simulink model "ROBOT_OK"  (R2021a)
settings: Solver=FixedStepAuto  StartTime=0.0  StopTime=inf  FixedStep=0.001  RelTol=1e-3
model workspace: external: MATLAB File E:\2024\TINH_TOAN_ROBOT_6_DOF\ROBOT_OK_DataFile.m (data not in the file)
values from neighbouring files (symbols this model uses):
  X = Toado(:,1)    [QuydaoK.m]
  Y = Toado(:,2)    [QuydaoK.m]
  Z = Toado(:,3)    [QuydaoK.m]
undefined symbols (not defined in the file or in its folder): smiData
libraries: sm_lib x38, nesl_utility x30, sharedutil x16, sharedtransform x12, dspmtrx3 x12, simulink_extras x8, pid_lib x6, simulink x3
(part 5 of 6)

== system ROBOT_OK/Subsystem2/Jacobian/J(q) gen./J_v_3(q)/J_v_1 ==
  R : Inport
  p : Inport  Port=2
  pn : Inport  Port=3
  type : Inport  Port=4
  Add : Sum
  If : If  IfExpression=u1 == 1
  Prismatic Action : Subsystem  TreatAsAtomicUnit=on
  Revolute Action : Subsystem  TreatAsAtomicUnit=on
  J_v : Outport
  wires:
  type/1 -> If/1
  If/1 -> Revolute Action/Action
  If/2 -> Prismatic Action/Action
  Revolute Action/1(J_v) -> Add/1
  Prismatic Action/1(J_v) -> Add/2
  Add/1 -> J_v/1
  R/1 -> Prismatic Action/1(R), Revolute Action/1(R)
  p/1 -> Revolute Action/2(p)
  pn/1 -> Revolute Action/3(pn)

== system ROBOT_OK/Subsystem2/Jacobian/J(q) gen./J_v_3(q)/J_v_2 ==
  R : Inport
  p : Inport  Port=2
  pn : Inport  Port=3
  type : Inport  Port=4
  Add : Sum
  If : If  IfExpression=u1 == 1
  Prismatic Action : Subsystem  TreatAsAtomicUnit=on
  Revolute Action : Subsystem  TreatAsAtomicUnit=on
  J_v : Outport
  wires:
  type/1 -> If/1
  If/1 -> Revolute Action/Action
  If/2 -> Prismatic Action/Action
  Revolute Action/1(J_v) -> Add/1
  Prismatic Action/1(J_v) -> Add/2
  Add/1 -> J_v/1
  R/1 -> Prismatic Action/1(R), Revolute Action/1(R)
  p/1 -> Revolute Action/2(p)
  pn/1 -> Revolute Action/3(pn)

== system ROBOT_OK/Subsystem2/Jacobian/J(q) gen./J_v_4(q)/J_v_1 ==
  R : Inport
  p : Inport  Port=2
  pn : Inport  Port=3
  type : Inport  Port=4
  Add : Sum
  If : If  IfExpression=u1 == 1
  Prismatic Action : Subsystem  TreatAsAtomicUnit=on
  Revolute Action : Subsystem  TreatAsAtomicUnit=on
  J_v : Outport
  wires:
  type/1 -> If/1
  If/1 -> Revolute Action/Action
  If/2 -> Prismatic Action/Action
  Revolute Action/1(J_v) -> Add/1
  Prismatic Action/1(J_v) -> Add/2
  Add/1 -> J_v/1
  R/1 -> Prismatic Action/1(R), Revolute Action/1(R)
  p/1 -> Revolute Action/2(p)
  pn/1 -> Revolute Action/3(pn)

== system ROBOT_OK/Subsystem2/Jacobian/J(q) gen./J_v_4(q)/J_v_2 ==
  R : Inport
  p : Inport  Port=2
  pn : Inport  Port=3
  type : Inport  Port=4
  Add : Sum
  If : If  IfExpression=u1 == 1
  Prismatic Action : Subsystem  TreatAsAtomicUnit=on
  Revolute Action : Subsystem  TreatAsAtomicUnit=on
  J_v : Outport
  wires:
  type/1 -> If/1
  If/1 -> Revolute Action/Action
  If/2 -> Prismatic Action/Action
  Revolute Action/1(J_v) -> Add/1
  Prismatic Action/1(J_v) -> Add/2
  Add/1 -> J_v/1
  R/1 -> Prismatic Action/1(R), Revolute Action/1(R)
  p/1 -> Revolute Action/2(p)
  pn/1 -> Revolute Action/3(pn)

== system ROBOT_OK/Subsystem2/Jacobian/J(q) gen./J_v_4(q)/J_v_3 ==
  R : Inport
  p : Inport  Port=2
  pn : Inport  Port=3
  type : Inport  Port=4
  Add : Sum
  If : If  IfExpression=u1 == 1
  Prismatic Action : Subsystem  TreatAsAtomicUnit=on
  Revolute Action : Subsystem  TreatAsAtomicUnit=on
  J_v : Outport
  wires:
  type/1 -> If/1
  If/1 -> Revolute Action/Action
  If/2 -> Prismatic Action/Action
  Revolute Action/1(J_v) -> Add/1
  Prismatic Action/1(J_v) -> Add/2
  Add/1 -> J_v/1
  R/1 -> Prismatic Action/1(R), Revolute Action/1(R)
  p/1 -> Revolute Action/2(p)
  pn/1 -> Revolute Action/3(pn)

== system ROBOT_OK/Subsystem2/Jacobian/J(q) gen./J_v_5(q)/J_v_1 ==
  R : Inport
  p : Inport  Port=2
  pn : Inport  Port=3
  type : Inport  Port=4
  Add : Sum
  If : If  IfExpression=u1 == 1
  Prismatic Action : Subsystem  TreatAsAtomicUnit=on
  Revolute Action : Subsystem  TreatAsAtomicUnit=on
  J_v : Outport
  wires:
  type/1 -> If/1
  If/1 -> Revolute Action/Action
  If/2 -> Prismatic Action/Action
  Revolute Action/1(J_v) -> Add/1
  Prismatic Action/1(J_v) -> Add/2
  Add/1 -> J_v/1
  R/1 -> Prismatic Action/1(R), Revolute Action/1(R)
  p/1 -> Revolute Action/2(p)
  pn/1 -> Revolute Action/3(pn)

== system ROBOT_OK/Subsystem2/Jacobian/J(q) gen./J_v_5(q)/J_v_2 ==
  R : Inport
  p : Inport  Port=2
  pn : Inport  Port=3
  type : Inport  Port=4
  Add : Sum
  If : If  IfExpression=u1 == 1
  Prismatic Action : Subsystem  TreatAsAtomicUnit=on
  Revolute Action : Subsystem  TreatAsAtomicUnit=on
  J_v : Outport
  wires:
  type/1 -> If/1
  If/1 -> Revolute Action/Action
  If/2 -> Prismatic Action/Action
  Revolute Action/1(J_v) -> Add/1
  Prismatic Action/1(J_v) -> Add/2
  Add/1 -> J_v/1
  R/1 -> Prismatic Action/1(R), Revolute Action/1(R)
  p/1 -> Revolute Action/2(p)
  pn/1 -> Revolute Action/3(pn)

== system ROBOT_OK/Subsystem2/Jacobian/J(q) gen./J_v_5(q)/J_v_3 ==
  R : Inport
  p : Inport  Port=2
  pn : Inport  Port=3
  type : Inport  Port=4
  Add : Sum
  If : If  IfExpression=u1 == 1
  Prismatic Action : Subsystem  TreatAsAtomicUnit=on
  Revolute Action : Subsystem  TreatAsAtomicUnit=on
  J_v : Outport
  wires:
  type/1 -> If/1
  If/1 -> Revolute Action/Action
  If/2 -> Prismatic Action/Action
  Revolute Action/1(J_v) -> Add/1
  Prismatic Action/1(J_v) -> Add/2
  Add/1 -> J_v/1
  R/1 -> Prismatic Action/1(R), Revolute Action/1(R)
  p/1 -> Revolute Action/2(p)
  pn/1 -> Revolute Action/3(pn)

== system ROBOT_OK/Subsystem2/Jacobian/J(q) gen./J_v_5(q)/J_v_4 ==
  R : Inport
  p : Inport  Port=2
  pn : Inport  Port=3
  type : Inport  Port=4
  Add : Sum
  If : If  IfExpression=u1 == 1
  Prismatic Action : Subsystem  TreatAsAtomicUnit=on
  Revolute Action : Subsystem  TreatAsAtomicUnit=on
  J_v : Outport
  wires:
  type/1 -> If/1
  If/1 -> Revolute Action/Action
  If/2 -> Prismatic Action/Action
  Revolute Action/1(J_v) -> Add/1
  Prismatic Action/1(J_v) -> Add/2
  Add/1 -> J_v/1
  R/1 -> Prismatic Action/1(R), Revolute Action/1(R)
  p/1 -> Revolute Action/2(p)
  pn/1 -> Revolute Action/3(pn)

== system ROBOT_OK/Subsystem2/Jacobian/J_v/J_v_1/Prismatic Action ==
  R : Inport
  Action Port : ActionPort  ActionPortLabel=else
  Constant : Constant  Value=[0;0;1]
  Product : Product  Multiplication=Matrix(*)
  J_v : Outport
  wires:
  Product/1 -> J_v/1
  R/1 -> Product/1
  Constant/1 -> Product/2

== system ROBOT_OK/Subsystem2/Jacobian/J_v/J_v_1/Revolute Action ==
  R : Inport
  p : Inport  Port=2
  pn : Inport  Port=3
  Action Port : ActionPort  ActionPortLabel=if(u1 == 1)
  3x3 Cross Product : sharedutil/3x3 Cross Product  aMode=aMode
      settings: SourceProductBaseCode=AE
  Add : Sum  Inputs=-+
  Constant : Constant  Value=[0;0;1]
  Product : Product  Multiplication=Matrix(*)
  J_v : Outport
  wires:
  3x3 Cross Product/1 -> J_v/1
  p/1 -> Add/1
  pn/1 -> Add/2
  Add/1 -> 3x3 Cross Product/2
  R/1 -> Product/1
  Constant/1 -> Product/2
  Product/1 -> 3x3 Cross Product/1

== system ROBOT_OK/Subsystem2/Jacobian/J_v/J_v_2/Prismatic Action ==
  R : Inport
  Action Port : ActionPort  ActionPortLabel=else
  Constant : Constant  Value=[0;0;1]
  Product : Product  Multiplication=Matrix(*)
  J_v : Outport
  wires:
  Product/1 -> J_v/1
  R/1 -> Product/1
  Constant/1 -> Product/2

== system ROBOT_OK/Subsystem2/Jacobian/J_v/J_v_2/Revolute Action ==
  R : Inport
  p : Inport  Port=2
  pn : Inport  Port=3
  Action Port : ActionPort  ActionPortLabel=if(u1 == 1)
  3x3 Cross Product : sharedutil/3x3 Cross Product  aMode=aMode
      settings: SourceProductBaseCode=AE
  Add : Sum  Inputs=-+
  Constant : Constant  Value=[0;0;1]
  Product : Product  Multiplication=Matrix(*)
  J_v : Outport
  wires:
  3x3 Cross Product/1 -> J_v/1
  p/1 -> Add/1
  pn/1 -> Add/2
  Add/1 -> 3x3 Cross Product/2
  R/1 -> Product/1
  Constant/1 -> Product/2
  Product/1 -> 3x3 Cross Product/1

== system ROBOT_OK/Subsystem2/Jacobian/J_v/J_v_3/Prismatic Action ==
  R : Inport
  Action Port : ActionPort  ActionPortLabel=else
  Constant : Constant  Value=[0;0;1]
  Product : Product  Multiplication=Matrix(*)
  J_v : Outport
  wires:
  Product/1 -> J_v/1
  R/1 -> Product/1
  Constant/1 -> Product/2

== system ROBOT_OK/Subsystem2/Jacobian/J_v/J_v_3/Revolute Action ==
  R : Inport
  p : Inport  Port=2
  pn : Inport  Port=3
  Action Port : ActionPort  ActionPortLabel=if(u1 == 1)
  3x3 Cross Product : sharedutil/3x3 Cross Product  aMode=aMode
      settings: SourceProductBaseCode=AE
  Add : Sum  Inputs=-+
  Constant : Constant  Value=[0;0;1]
  Product : Product  Multiplication=Matrix(*)
  J_v : Outport
  wires:
  3x3 Cross Product/1 -> J_v/1
  p/1 -> Add/1
  pn/1 -> Add/2
  Add/1 -> 3x3 Cross Product/2
  R/1 -> Product/1
  Constant/1 -> Product/2
  Product/1 -> 3x3 Cross Product/1

== system ROBOT_OK/Subsystem2/Jacobian/J_v/J_v_4/Prismatic Action ==
  R : Inport
  Action Port : ActionPort  ActionPortLabel=else
  Constant : Constant  Value=[0;0;1]
  Product : Product  Multiplication=Matrix(*)
  J_v : Outport
  wires:
  Product/1 -> J_v/1
  R/1 -> Product/1
  Constant/1 -> Product/2

== system ROBOT_OK/Subsystem2/Jacobian/J_v/J_v_4/Revolute Action ==
  R : Inport
  p : Inport  Port=2
  pn : Inport  Port=3
  Action Port : ActionPort  ActionPortLabel=if(u1 == 1)
  3x3 Cross Product : sharedutil/3x3 Cross Product  aMode=aMode
      settings: SourceProductBaseCode=AE
  Add : Sum  Inputs=-+
  Constant : Constant  Value=[0;0;1]
  Product : Product  Multiplication=Matrix(*)
  J_v : Outport
  wires:
  3x3 Cross Product/1 -> J_v/1
  p/1 -> Add/1
  pn/1 -> Add/2
  Add/1 -> 3x3 Cross Product/2
  R/1 -> Product/1
  Constant/1 -> Product/2
  Product/1 -> 3x3 Cross Product/1

== system ROBOT_OK/Subsystem2/Jacobian/J_v/J_v_5/Prismatic Action ==
  R : Inport
  Action Port : ActionPort  ActionPortLabel=else
  Constant : Constant  Value=[0;0;1]
  Product : Product  Multiplication=Matrix(*)
  J_v : Outport
  wires:
  Product/1 -> J_v/1
  R/1 -> Product/1
  Constant/1 -> Product/2

== system ROBOT_OK/Subsystem2/Jacobian/J_v/J_v_5/Revolute Action ==
  R : Inport
  p : Inport  Port=2
  pn : Inport  Port=3
  Action Port : ActionPort  ActionPortLabel=if(u1 == 1)
  3x3 Cross Product : sharedutil/3x3 Cross Product  aMode=aMode
      settings: SourceProductBaseCode=AE
  Add : Sum  Inputs=-+
  Constant : Constant  Value=[0;0;1]
  Product : Product  Multiplication=Matrix(*)
  J_v : Outport
  wires:
  3x3 Cross Product/1 -> J_v/1
  p/1 -> Add/1
  pn/1 -> Add/2
  Add/1 -> 3x3 Cross Product/2
  R/1 -> Product/1
  Constant/1 -> Product/2
  Product/1 -> 3x3 Cross Product/1

== system ROBOT_OK/Subsystem2/Jacobian/J_v/J_v_6/Prismatic Action ==
  R : Inport
  Action Port : ActionPort  ActionPortLabel=else
  Constant : Constant  Value=[0;0;1]
  Product : Product  Multiplication=Matrix(*)
  J_v : Outport
  wires:
  Product/1 -> J_v/1
  R/1 -> Product/1
  Constant/1 -> Product/2

== system ROBOT_OK/Subsystem2/Jacobian/J_v/J_v_6/Revolute Action ==
  R : Inport
  p : Inport  Port=2
  pn : Inport  Port=3
  Action Port : ActionPort  ActionPortLabel=if(u1 == 1)
  3x3 Cross Product : sharedutil/3x3 Cross Product  aMode=aMode
      settings: SourceProductBaseCode=AE
  Add : Sum  Inputs=-+
  Constant : Constant  Value=[0;0;1]
  Product : Product  Multiplication=Matrix(*)
  J_v : Outport
  wires:
  3x3 Cross Product/1 -> J_v/1
  p/1 -> Add/1
  pn/1 -> Add/2
  Add/1 -> 3x3 Cross Product/2
  R/1 -> Product/1
  Constant/1 -> Product/2
  Product/1 -> 3x3 Cross Product/1

== system ROBOT_OK/Động Lực Học2/Jacobian/J(q) gen./J_v_2(q)/J_v_1 ==
  R : Inport
  p : Inport  Port=2
  pn : Inport  Port=3
  type : Inport  Port=4
  Add : Sum
  If : If  IfExpression=u1 == 1
  Prismatic Action : Subsystem  TreatAsAtomicUnit=on
  Revolute Action : Subsystem  TreatAsAtomicUnit=on
  J_v : Outport
  wires:
  type/1 -> If/1
  If/1 -> Revolute Action/Action
  If/2 -> Prismatic Action/Action
  Revolute Action/1(J_v) -> Add/1
  Prismatic Action/1(J_v) -> Add/2
  Add/1 -> J_v/1
  R/1 -> Prismatic Action/1(R), Revolute Action/1(R)
  p/1 -> Revolute Action/2(p)
  pn/1 -> Revolute Action/3(pn)

== system ROBOT_OK/Động Lực Học2/Jacobian/J(q) gen./J_v_3(q)/J_v_1 ==
  R : Inport
  p : Inport  Port=2
  pn : Inport  Port=3
  type : Inport  Port=4
  Add : Sum
  If : If  IfExpression=u1 == 1
  Prismatic Action : Subsystem  TreatAsAtomicUnit=on
  Revolute Action : Subsystem  TreatAsAtomicUnit=on
  J_v : Outport
  wires:
  type/1 -> If/1
  If/1 -> Revolute Action/Action
  If/2 -> Prismatic Action/Action
  Revolute Action/1(J_v) -> Add/1
  Prismatic Action/1(J_v) -> Add/2
  Add/1 -> J_v/1
  R/1 -> Prismatic Action/1(R), Revolute Action/1(R)
  p/1 -> Revolute Action/2(p)
  pn/1 -> Revolute Action/3(pn)

== system ROBOT_OK/Động Lực Học2/Jacobian/J(q) gen./J_v_3(q)/J_v_2 ==
  R : Inport
  p : Inport  Port=2
  pn : Inport  Port=3
  type : Inport  Port=4
  Add : Sum
  If : If  IfExpression=u1 == 1
  Prismatic Action : Subsystem  TreatAsAtomicUnit=on
  Revolute Action : Subsystem  TreatAsAtomicUnit=on
  J_v : Outport
  wires:
  type/1 -> If/1
  If/1 -> Revolute Action/Action
  If/2 -> Prismatic Action/Action
  Revolute Action/1(J_v) -> Add/1
  Prismatic Action/1(J_v) -> Add/2
  Add/1 -> J_v/1
  R/1 -> Prismatic Action/1(R), Revolute Action/1(R)
  p/1 -> Revolute Action/2(p)
  pn/1 -> Revolute Action/3(pn)

== system ROBOT_OK/Động Lực Học2/Jacobian/J(q) gen./J_v_4(q)/J_v_1 ==
  R : Inport
  p : Inport  Port=2
  pn : Inport  Port=3
  type : Inport  Port=4
  Add : Sum
  If : If  IfExpression=u1 == 1
  Prismatic Action : Subsystem  TreatAsAtomicUnit=on
  Revolute Action : Subsystem  TreatAsAtomicUnit=on
  J_v : Outport
  wires:
  type/1 -> If/1
  If/1 -> Revolute Action/Action
  If/2 -> Prismatic Action/Action
  Revolute Action/1(J_v) -> Add/1
  Prismatic Action/1(J_v) -> Add/2
  Add/1 -> J_v/1
  R/1 -> Prismatic Action/1(R), Revolute Action/1(R)
  p/1 -> Revolute Action/2(p)
  pn/1 -> Revolute Action/3(pn)

== system ROBOT_OK/Động Lực Học2/Jacobian/J(q) gen./J_v_4(q)/J_v_2 ==
  R : Inport
  p : Inport  Port=2
  pn : Inport  Port=3
  type : Inport  Port=4
  Add : Sum
  If : If  IfExpression=u1 == 1
  Prismatic Action : Subsystem  TreatAsAtomicUnit=on
  Revolute Action : Subsystem  TreatAsAtomicUnit=on
  J_v : Outport
  wires:
  type/1 -> If/1
  If/1 -> Revolute Action/Action
  If/2 -> Prismatic Action/Action
  Revolute Action/1(J_v) -> Add/1
  Prismatic Action/1(J_v) -> Add/2
  Add/1 -> J_v/1
  R/1 -> Prismatic Action/1(R), Revolute Action/1(R)
  p/1 -> Revolute Action/2(p)
  pn/1 -> Revolute Action/3(pn)

== system ROBOT_OK/Động Lực Học2/Jacobian/J(q) gen./J_v_4(q)/J_v_3 ==
  R : Inport
  p : Inport  Port=2
  pn : Inport  Port=3
  type : Inport  Port=4
  Add : Sum
  If : If  IfExpression=u1 == 1
  Prismatic Action : Subsystem  TreatAsAtomicUnit=on
  Revolute Action : Subsystem  TreatAsAtomicUnit=on
  J_v : Outport
  wires:
  type/1 -> If/1
  If/1 -> Revolute Action/Action
  If/2 -> Prismatic Action/Action
  Revolute Action/1(J_v) -> Add/1
  Prismatic Action/1(J_v) -> Add/2
  Add/1 -> J_v/1
  R/1 -> Prismatic Action/1(R), Revolute Action/1(R)
  p/1 -> Revolute Action/2(p)
  pn/1 -> Revolute Action/3(pn)

== system ROBOT_OK/Động Lực Học2/Jacobian/J(q) gen./J_v_5(q)/J_v_1 ==
  R : Inport
  p : Inport  Port=2
  pn : Inport  Port=3
  type : Inport  Port=4
  Add : Sum
  If : If  IfExpression=u1 == 1
  Prismatic Action : Subsystem  TreatAsAtomicUnit=on
  Revolute Action : Subsystem  TreatAsAtomicUnit=on
  J_v : Outport
  wires:
  type/1 -> If/1
  If/1 -> Revolute Action/Action
  If/2 -> Prismatic Action/Action
  Revolute Action/1(J_v) -> Add/1
  Prismatic Action/1(J_v) -> Add/2
  Add/1 -> J_v/1
  R/1 -> Prismatic Action/1(R), Revolute Action/1(R)
  p/1 -> Revolute Action/2(p)
  pn/1 -> Revolute Action/3(pn)

== system ROBOT_OK/Động Lực Học2/Jacobian/J(q) gen./J_v_5(q)/J_v_2 ==
  R : Inport
  p : Inport  Port=2
  pn : Inport  Port=3
  type : Inport  Port=4
  Add : Sum
  If : If  IfExpression=u1 == 1
  Prismatic Action : Subsystem  TreatAsAtomicUnit=on
  Revolute Action : Subsystem  TreatAsAtomicUnit=on
  J_v : Outport
  wires:
  type/1 -> If/1
  If/1 -> Revolute Action/Action
  If/2 -> Prismatic Action/Action
  Revolute Action/1(J_v) -> Add/1
  Prismatic Action/1(J_v) -> Add/2
  Add/1 -> J_v/1
  R/1 -> Prismatic Action/1(R), Revolute Action/1(R)
  p/1 -> Revolute Action/2(p)
  pn/1 -> Revolute Action/3(pn)

== system ROBOT_OK/Động Lực Học2/Jacobian/J(q) gen./J_v_5(q)/J_v_3 ==
  R : Inport
  p : Inport  Port=2
  pn : Inport  Port=3
  type : Inport  Port=4
  Add : Sum
  If : If  IfExpression=u1 == 1
  Prismatic Action : Subsystem  TreatAsAtomicUnit=on
  Revolute Action : Subsystem  TreatAsAtomicUnit=on
  J_v : Outport
  wires:
  type/1 -> If/1
  If/1 -> Revolute Action/Action
  If/2 -> Prismatic Action/Action
  Revolute Action/1(J_v) -> Add/1
  Prismatic Action/1(J_v) -> Add/2
  Add/1 -> J_v/1
  R/1 -> Prismatic Action/1(R), Revolute Action/1(R)
  p/1 -> Revolute Action/2(p)
  pn/1 -> Revolute Action/3(pn)

== system ROBOT_OK/Động Lực Học2/Jacobian/J(q) gen./J_v_5(q)/J_v_4 ==
  R : Inport
  p : Inport  Port=2
  pn : Inport  Port=3
  type : Inport  Port=4
  Add : Sum
  If : If  IfExpression=u1 == 1
  Prismatic Action : Subsystem  TreatAsAtomicUnit=on
  Revolute Action : Subsystem  TreatAsAtomicUnit=on
  J_v : Outport
  wires:
  type/1 -> If/1
  If/1 -> Revolute Action/Action
  If/2 -> Prismatic Action/Action
  Revolute Action/1(J_v) -> Add/1
  Prismatic Action/1(J_v) -> Add/2
  Add/1 -> J_v/1
  R/1 -> Prismatic Action/1(R), Revolute Action/1(R)
  p/1 -> Revolute Action/2(p)
  pn/1 -> Revolute Action/3(pn)

== system ROBOT_OK/Động Lực Học2/Jacobian/J_v/J_v_1/Prismatic Action ==
  R : Inport
  Action Port : ActionPort
  Constant : Constant  Value=[0;0;1]
  Product : Product  Multiplication=Matrix(*)
  J_v : Outport
  wires:
  Product/1 -> J_v/1
  R/1 -> Product/1
  Constant/1 -> Product/2

== system ROBOT_OK/Động Lực Học2/Jacobian/J_v/J_v_1/Revolute Action ==
  R : Inport
  p : Inport  Port=2
  pn : Inport  Port=3
  Action Port : ActionPort
  3x3 Cross Product : Subsystem  Description=Replaced Block  mask(Replaced Block){}
      mask help: This block has been replaced with an empty subsystem because it used functionality that is unavailable in Simulink R2021a.
      mask Display: fprintf('Replaced: %s\n','CrossProduct')
  Add : Sum  Inputs=-+
  Constant : Constant  Value=[0;0;1]
  Product : Product  Multiplication=Matrix(*)
  J_v : Outport
  wires:
  3x3 Cross Product/1(Out1) -> J_v/1
  p/1 -> Add/1
  pn/1 -> Add/2
  Add/1 -> 3x3 Cross Product/2(In2)
  R/1 -> Product/1
  Constant/1 -> Product/2
  Product/1 -> 3x3 Cross Product/1(In1)

== system ROBOT_OK/Động Lực Học2/Jacobian/J_v/J_v_2/Prismatic Action ==
  R : Inport
  Action Port : ActionPort
  Constant : Constant  Value=[0;0;1]
  Product : Product  Multiplication=Matrix(*)
  J_v : Outport
  wires:
  Product/1 -> J_v/1
  R/1 -> Product/1
  Constant/1 -> Product/2

== system ROBOT_OK/Động Lực Học2/Jacobian/J_v/J_v_2/Revolute Action ==
  R : Inport
  p : Inport  Port=2
  pn : Inport  Port=3
  Action Port : ActionPort
  3x3 Cross Product : Subsystem  Description=Replaced Block  mask(Replaced Block){}
      mask help: This block has been replaced with an empty subsystem because it used functionality that is unavailable in Simulink R2021a.
      mask Display: fprintf('Replaced: %s\n','CrossProduct')
  Add : Sum  Inputs=-+
  Constant : Constant  Value=[0;0;1]
  Product : Product  Multiplication=Matrix(*)
  J_v : Outport
  wires:
  3x3 Cross Product/1(Out1) -> J_v/1
  p/1 -> Add/1
  pn/1 -> Add/2
  Add/1 -> 3x3 Cross Product/2(In2)
  R/1 -> Product/1
  Constant/1 -> Product/2
  Product/1 -> 3x3 Cross Product/1(In1)

== system ROBOT_OK/Động Lực Học2/Jacobian/J_v/J_v_3/Prismatic Action ==
  R : Inport
  Action Port : ActionPort
  Constant : Constant  Value=[0;0;1]
  Product : Product  Multiplication=Matrix(*)
  J_v : Outport
  wires:
  Product/1 -> J_v/1
  R/1 -> Product/1
  Constant/1 -> Product/2

== system ROBOT_OK/Động Lực Học2/Jacobian/J_v/J_v_3/Revolute Action ==
  R : Inport
  p : Inport  Port=2
  pn : Inport  Port=3
  Action Port : ActionPort
  3x3 Cross Product : Subsystem  Description=Replaced Block  mask(Replaced Block){}
      mask help: This block has been replaced with an empty subsystem because it used functionality that is unavailable in Simulink R2021a.
      mask Display: fprintf('Replaced: %s\n','CrossProduct')
  Add : Sum  Inputs=-+
  Constant : Constant  Value=[0;0;1]
  Product : Product  Multiplication=Matrix(*)
  J_v : Outport
  wires:
  3x3 Cross Product/1(Out1) -> J_v/1
  p/1 -> Add/1
  pn/1 -> Add/2
  Add/1 -> 3x3 Cross Product/2(In2)
  R/1 -> Product/1
  Constant/1 -> Product/2
  Product/1 -> 3x3 Cross Product/1(In1)

== system ROBOT_OK/Động Lực Học2/Jacobian/J_v/J_v_4/Prismatic Action ==
  R : Inport
  Action Port : ActionPort
  Constant : Constant  Value=[0;0;1]
  Product : Product  Multiplication=Matrix(*)
  J_v : Outport
  wires:
  Product/1 -> J_v/1
  R/1 -> Product/1
  Constant/1 -> Product/2

== system ROBOT_OK/Động Lực Học2/Jacobian/J_v/J_v_4/Revolute Action ==
  R : Inport
  p : Inport  Port=2
  pn : Inport  Port=3
  Action Port : ActionPort
  3x3 Cross Product : Subsystem  Description=Replaced Block  mask(Replaced Block){}
      mask help: This block has been replaced with an empty subsystem because it used functionality that is unavailable in Simulink R2021a.
      mask Display: fprintf('Replaced: %s\n','CrossProduct')
  Add : Sum  Inputs=-+
  Constant : Constant  Value=[0;0;1]
  Product : Product  Multiplication=Matrix(*)
  J_v : Outport
  wires:
  3x3 Cross Product/1(Out1) -> J_v/1
  p/1 -> Add/1
  pn/1 -> Add/2
  Add/1 -> 3x3 Cross Product/2(In2)
  R/1 -> Product/1
  Constant/1 -> Product/2
  Product/1 -> 3x3 Cross Product/1(In1)

== system ROBOT_OK/Động Lực Học2/Jacobian/J_v/J_v_5/Prismatic Action ==
  R : Inport
  Action Port : ActionPort
  Constant : Constant  Value=[0;0;1]
  Product : Product  Multiplication=Matrix(*)
  J_v : Outport
  wires:
  Product/1 -> J_v/1
  R/1 -> Product/1
  Constant/1 -> Product/2

== system ROBOT_OK/Động Lực Học2/Jacobian/J_v/J_v_5/Revolute Action ==
  R : Inport
  p : Inport  Port=2
  pn : Inport  Port=3
  Action Port : ActionPort
  3x3 Cross Product : Subsystem  Description=Replaced Block  mask(Replaced Block){}
      mask help: This block has been replaced with an empty subsystem because it used functionality that is unavailable in Simulink R2021a.
      mask Display: fprintf('Replaced: %s\n','CrossProduct')
  Add : Sum  Inputs=-+
  Constant : Constant  Value=[0;0;1]
  Product : Product  Multiplication=Matrix(*)
  J_v : Outport
  wires:
  3x3 Cross Product/1(Out1) -> J_v/1
  p/1 -> Add/1
  pn/1 -> Add/2
  Add/1 -> 3x3 Cross Product/2(In2)
  R/1 -> Product/1
  Constant/1 -> Product/2
  Product/1 -> 3x3 Cross Product/1(In1)

== system ROBOT_OK/Động Lực Học2/Jacobian/J_v/J_v_6/Prismatic Action ==
  R : Inport
  Action Port : ActionPort
  Constant : Constant  Value=[0;0;1]
  Product : Product  Multiplication=Matrix(*)
  J_v : Outport
  wires:
  Product/1 -> J_v/1
  R/1 -> Product/1
  Constant/1 -> Product/2

== system ROBOT_OK/Động Lực Học2/Jacobian/J_v/J_v_6/Revolute Action ==
  R : Inport
  p : Inport  Port=2
  pn : Inport  Port=3
  Action Port : ActionPort
  3x3 Cross Product : Subsystem  Description=Replaced Block  mask(Replaced Block){}
      mask help: This block has been replaced with an empty subsystem because it used functionality that is unavailable in Simulink R2021a.
      mask Display: fprintf('Replaced: %s\n','CrossProduct')
  Add : Sum  Inputs=-+
  Constant : Constant  Value=[0;0;1]
  Product : Product  Multiplication=Matrix(*)
  J_v : Outport
  wires:
  3x3 Cross Product/1(Out1) -> J_v/1
  p/1 -> Add/1
  pn/1 -> Add/2
  Add/1 -> 3x3 Cross Product/2(In2)
  R/1 -> Product/1
  Constant/1 -> Product/2
  Product/1 -> 3x3 Cross Product/1(In1)

== system ROBOT_OK/Subsystem2/Jacobian/J(q) gen./J_v_2(q)/J_v_1/Prismatic Action ==
  R : Inport
  Action Port : ActionPort  ActionPortLabel=else
  Constant : Constant  Value=[0;0;1]
  Product : Product  Multiplication=Matrix(*)
  J_v : Outport
  wires:
  Product/1 -> J_v/1
  R/1 -> Product/1
  Constant/1 -> Product/2

== system ROBOT_OK/Subsystem2/Jacobian/J(q) gen./J_v_2(q)/J_v_1/Revolute Action ==
  R : Inport
  p : Inport  Port=2
  pn : Inport  Port=3
  Action Port : ActionPort  ActionPortLabel=if(u1 == 1)
  3x3 Cross Product : sharedutil/3x3 Cross Product  aMode=aMode
      settings: SourceProductBaseCode=AE
  Add : Sum  Inputs=-+
  Constant : Constant  Value=[0;0;1]
  Product : Product  Multiplication=Matrix(*)
  J_v : Outport
  wires:
  3x3 Cross Product/1 -> J_v/1
  p/1 -> Add/1
  pn/1 -> Add/2
  Add/1 -> 3x3 Cross Product/2
  R/1 -> Product/1
  Constant/1 -> Product/2
  Product/1 -> 3x3 Cross Product/1

== system ROBOT_OK/Subsystem2/Jacobian/J(q) gen./J_v_3(q)/J_v_1/Prismatic Action ==
  R : Inport
  Action Port : ActionPort  ActionPortLabel=else
  Constant : Constant  Value=[0;0;1]
  Product : Product  Multiplication=Matrix(*)
  J_v : Outport
  wires:
  Product/1 -> J_v/1
  R/1 -> Product/1
  Constant/1 -> Product/2

== system ROBOT_OK/Subsystem2/Jacobian/J(q) gen./J_v_3(q)/J_v_1/Revolute Action ==
  R : Inport
  p : Inport  Port=2
  pn : Inport  Port=3
  Action Port : ActionPort  ActionPortLabel=if(u1 == 1)
  3x3 Cross Product : sharedutil/3x3 Cross Product  aMode=aMode
      settings: SourceProductBaseCode=AE
  Add : Sum  Inputs=-+
  Constant : Constant  Value=[0;0;1]
  Product : Product  Multiplication=Matrix(*)
  J_v : Outport
  wires:
  3x3 Cross Product/1 -> J_v/1
  p/1 -> Add/1
  pn/1 -> Add/2
  Add/1 -> 3x3 Cross Product/2
  R/1 -> Product/1
  Constant/1 -> Product/2
  Product/1 -> 3x3 Cross Product/1

== system ROBOT_OK/Subsystem2/Jacobian/J(q) gen./J_v_3(q)/J_v_2/Prismatic Action ==
  R : Inport
  Action Port : ActionPort  ActionPortLabel=else
  Constant : Constant  Value=[0;0;1]
  Product : Product  Multiplication=Matrix(*)
  J_v : Outport
  wires:
  Product/1 -> J_v/1
  R/1 -> Product/1
  Constant/1 -> Product/2

== system ROBOT_OK/Subsystem2/Jacobian/J(q) gen./J_v_3(q)/J_v_2/Revolute Action ==
  R : Inport
  p : Inport  Port=2
  pn : Inport  Port=3
  Action Port : ActionPort  ActionPortLabel=if(u1 == 1)
  3x3 Cross Product : sharedutil/3x3 Cross Product  aMode=aMode
      settings: SourceProductBaseCode=AE
  Add : Sum  Inputs=-+
  Constant : Constant  Value=[0;0;1]
  Product : Product  Multiplication=Matrix(*)
  J_v : Outport
  wires:
  3x3 Cross Product/1 -> J_v/1
  p/1 -> Add/1
  pn/1 -> Add/2
  Add/1 -> 3x3 Cross Product/2
  R/1 -> Product/1
  Constant/1 -> Product/2
  Product/1 -> 3x3 Cross Product/1

== system ROBOT_OK/Subsystem2/Jacobian/J(q) gen./J_v_4(q)/J_v_1/Prismatic Action ==
  R : Inport
  Action Port : ActionPort  ActionPortLabel=else
  Constant : Constant  Value=[0;0;1]
  Product : Product  Multiplication=Matrix(*)
  J_v : Outport
  wires:
  Product/1 -> J_v/1
  R/1 -> Product/1
  Constant/1 -> Product/2

== system ROBOT_OK/Subsystem2/Jacobian/J(q) gen./J_v_4(q)/J_v_1/Revolute Action ==
  R : Inport
  p : Inport  Port=2
  pn : Inport  Port=3
  Action Port : ActionPort  ActionPortLabel=if(u1 == 1)
  3x3 Cross Product : sharedutil/3x3 Cross Product  aMode=aMode
      settings: SourceProductBaseCode=AE
  Add : Sum  Inputs=-+
  Constant : Constant  Value=[0;0;1]
  Product : Product  Multiplication=Matrix(*)
  J_v : Outport
  wires:
  3x3 Cross Product/1 -> J_v/1
  p/1 -> Add/1
  pn/1 -> Add/2
  Add/1 -> 3x3 Cross Product/2
  R/1 -> Product/1
  Constant/1 -> Product/2
  Product/1 -> 3x3 Cross Product/1

== system ROBOT_OK/Subsystem2/Jacobian/J(q) gen./J_v_4(q)/J_v_2/Prismatic Action ==
  R : Inport
  Action Port : ActionPort  ActionPortLabel=else
  Constant : Constant  Value=[0;0;1]
  Product : Product  Multiplication=Matrix(*)
  J_v : Outport
  wires:
  Product/1 -> J_v/1
  R/1 -> Product/1
  Constant/1 -> Product/2

== system ROBOT_OK/Subsystem2/Jacobian/J(q) gen./J_v_4(q)/J_v_2/Revolute Action ==
  R : Inport
  p : Inport  Port=2
  pn : Inport  Port=3
  Action Port : ActionPort  ActionPortLabel=if(u1 == 1)
  3x3 Cross Product : sharedutil/3x3 Cross Product  aMode=aMode
      settings: SourceProductBaseCode=AE
  Add : Sum  Inputs=-+
  Constant : Constant  Value=[0;0;1]
  Product : Product  Multiplication=Matrix(*)
  J_v : Outport
  wires:
  3x3 Cross Product/1 -> J_v/1
  p/1 -> Add/1
  pn/1 -> Add/2
  Add/1 -> 3x3 Cross Product/2
  R/1 -> Product/1
  Constant/1 -> Product/2
  Product/1 -> 3x3 Cross Product/1

== system ROBOT_OK/Subsystem2/Jacobian/J(q) gen./J_v_4(q)/J_v_3/Prismatic Action ==
  R : Inport
  Action Port : ActionPort  ActionPortLabel=else
  Constant : Constant  Value=[0;0;1]
  Product : Product  Multiplication=Matrix(*)
  J_v : Outport
  wires:
  Product/1 -> J_v/1
  R/1 -> Product/1
  Constant/1 -> Product/2

== system ROBOT_OK/Subsystem2/Jacobian/J(q) gen./J_v_4(q)/J_v_3/Revolute Action ==
  R : Inport
  p : Inport  Port=2
  pn : Inport  Port=3
  Action Port : ActionPort  ActionPortLabel=if(u1 == 1)
  3x3 Cross Product : sharedutil/3x3 Cross Product  aMode=aMode
      settings: SourceProductBaseCode=AE
  Add : Sum  Inputs=-+
  Constant : Constant  Value=[0;0;1]
  Product : Product  Multiplication=Matrix(*)
  J_v : Outport
  wires:
  3x3 Cross Product/1 -> J_v/1
  p/1 -> Add/1
  pn/1 -> Add/2
  Add/1 -> 3x3 Cross Product/2
  R/1 -> Product/1
  Constant/1 -> Product/2
  Product/1 -> 3x3 Cross Product/1

== system ROBOT_OK/Subsystem2/Jacobian/J(q) gen./J_v_5(q)/J_v_1/Prismatic Action ==
  R : Inport
  Action Port : ActionPort  ActionPortLabel=else
  Constant : Constant  Value=[0;0;1]
  Product : Product  Multiplication=Matrix(*)
  J_v : Outport
  wires:
  Product/1 -> J_v/1
  R/1 -> Product/1
  Constant/1 -> Product/2

== system ROBOT_OK/Subsystem2/Jacobian/J(q) gen./J_v_5(q)/J_v_1/Revolute Action ==
  R : Inport
  p : Inport  Port=2
  pn : Inport  Port=3
  Action Port : ActionPort  ActionPortLabel=if(u1 == 1)
  3x3 Cross Product : sharedutil/3x3 Cross Product  aMode=aMode
      settings: SourceProductBaseCode=AE
  Add : Sum  Inputs=-+
  Constant : Constant  Value=[0;0;1]
  Product : Product  Multiplication=Matrix(*)
  J_v : Outport
  wires:
  3x3 Cross Product/1 -> J_v/1
  p/1 -> Add/1
  pn/1 -> Add/2
  Add/1 -> 3x3 Cross Product/2
  R/1 -> Product/1
  Constant/1 -> Product/2
  Product/1 -> 3x3 Cross Product/1

== system ROBOT_OK/Subsystem2/Jacobian/J(q) gen./J_v_5(q)/J_v_2/Prismatic Action ==
  R : Inport
  Action Port : ActionPort  ActionPortLabel=else
  Constant : Constant  Value=[0;0;1]
  Product : Product  Multiplication=Matrix(*)
  J_v : Outport
  wires:
  Product/1 -> J_v/1
  R/1 -> Product/1
  Constant/1 -> Product/2

== system ROBOT_OK/Subsystem2/Jacobian/J(q) gen./J_v_5(q)/J_v_2/Revolute Action ==
  R : Inport
  p : Inport  Port=2
  pn : Inport  Port=3
  Action Port : ActionPort  ActionPortLabel=if(u1 == 1)
  3x3 Cross Product : sharedutil/3x3 Cross Product  aMode=aMode
      settings: SourceProductBaseCode=AE
  Add : Sum  Inputs=-+
  Constant : Constant  Value=[0;0;1]
  Product : Product  Multiplication=Matrix(*)
  J_v : Outport
  wires:
  3x3 Cross Product/1 -> J_v/1
  p/1 -> Add/1
  pn/1 -> Add/2
  Add/1 -> 3x3 Cross Product/2
  R/1 -> Product/1
  Constant/1 -> Product/2
  Product/1 -> 3x3 Cross Product/1

== system ROBOT_OK/Subsystem2/Jacobian/J(q) gen./J_v_5(q)/J_v_3/Prismatic Action ==
  R : Inport
  Action Port : ActionPort  ActionPortLabel=else
  Constant : Constant  Value=[0;0;1]
  Product : Product  Multiplication=Matrix(*)
  J_v : Outport
  wires:
  Product/1 -> J_v/1
  R/1 -> Product/1
  Constant/1 -> Product/2

== system ROBOT_OK/Subsystem2/Jacobian/J(q) gen./J_v_5(q)/J_v_3/Revolute Action ==
  R : Inport
  p : Inport  Port=2
  pn : Inport  Port=3
  Action Port : ActionPort  ActionPortLabel=if(u1 == 1)
  3x3 Cross Product : sharedutil/3x3 Cross Product  aMode=aMode
      settings: SourceProductBaseCode=AE
  Add : Sum  Inputs=-+
  Constant : Constant  Value=[0;0;1]
  Product : Product  Multiplication=Matrix(*)
  J_v : Outport
  wires:
  3x3 Cross Product/1 -> J_v/1
  p/1 -> Add/1
  pn/1 -> Add/2
  Add/1 -> 3x3 Cross Product/2
  R/1 -> Product/1
  Constant/1 -> Product/2
  Product/1 -> 3x3 Cross Product/1

== system ROBOT_OK/Subsystem2/Jacobian/J(q) gen./J_v_5(q)/J_v_4/Prismatic Action ==
  R : Inport
  Action Port : ActionPort  ActionPortLabel=else
  Constant : Constant  Value=[0;0;1]
  Product : Product  Multiplication=Matrix(*)
  J_v : Outport
  wires:
  Product/1 -> J_v/1
  R/1 -> Product/1
  Constant/1 -> Product/2

== system ROBOT_OK/Subsystem2/Jacobian/J(q) gen./J_v_5(q)/J_v_4/Revolute Action ==
  R : Inport
  p : Inport  Port=2
  pn : Inport  Port=3
  Action Port : ActionPort  ActionPortLabel=if(u1 == 1)
  3x3 Cross Product : sharedutil/3x3 Cross Product  aMode=aMode
      settings: SourceProductBaseCode=AE
  Add : Sum  Inputs=-+
  Constant : Constant  Value=[0;0;1]
  Product : Product  Multiplication=Matrix(*)
  J_v : Outport
  wires:
  3x3 Cross Product/1 -> J_v/1
  p/1 -> Add/1
  pn/1 -> Add/2
  Add/1 -> 3x3 Cross Product/2
  R/1 -> Product/1
  Constant/1 -> Product/2
  Product/1 -> 3x3 Cross Product/1

== system ROBOT_OK/Động Lực Học2/Jacobian/J(q) gen./J_v_2(q)/J_v_1/Prismatic Action ==
  R : Inport
  Action Port : ActionPort
  Constant : Constant  Value=[0;0;1]
  Product : Product  Multiplication=Matrix(*)
  J_v : Outport
  wires:
  Product/1 -> J_v/1
  R/1 -> Product/1
  Constant/1 -> Product/2

== system ROBOT_OK/Động Lực Học2/Jacobian/J(q) gen./J_v_2(q)/J_v_1/Revolute Action ==
  R : Inport
  p : Inport  Port=2
  pn : Inport  Port=3
  Action Port : ActionPort
  3x3 Cross Product : Subsystem  Description=Replaced Block  mask(Replaced Block){}
      mask help: This block has been replaced with an empty subsystem because it used functionality that is unavailable in Simulink R2021a.
      mask Display: fprintf('Replaced: %s\n','CrossProduct')
  Add : Sum  Inputs=-+
  Constant : Constant  Value=[0;0;1]
  Product : Product  Multiplication=Matrix(*)
  J_v : Outport
  wires:
  3x3 Cross Product/1(Out1) -> J_v/1
  p/1 -> Add/1
  pn/1 -> Add/2
  Add/1 -> 3x3 Cross Product/2(In2)
  R/1 -> Product/1
  Constant/1 -> Product/2
  Product/1 -> 3x3 Cross Product/1(In1)

== system ROBOT_OK/Động Lực Học2/Jacobian/J(q) gen./J_v_3(q)/J_v_1/Prismatic Action ==
  R : Inport
  Action Port : ActionPort
  Constant : Constant  Value=[0;0;1]
  Product : Product  Multiplication=Matrix(*)
  J_v : Outport
  wires:
  Product/1 -> J_v/1
  R/1 -> Product/1
  Constant/1 -> Product/2

== system ROBOT_OK/Động Lực Học2/Jacobian/J(q) gen./J_v_3(q)/J_v_1/Revolute Action ==
  R : Inport
  p : Inport  Port=2
  pn : Inport  Port=3
  Action Port : ActionPort
  3x3 Cross Product : Subsystem  Description=Replaced Block  mask(Replaced Block){}
      mask help: This block has been replaced with an empty subsystem because it used functionality that is unavailable in Simulink R2021a.
      mask Display: fprintf('Replaced: %s\n','CrossProduct')
  Add : Sum  Inputs=-+
  Constant : Constant  Value=[0;0;1]
  Product : Product  Multiplication=Matrix(*)
  J_v : Outport
  wires:
  3x3 Cross Product/1(Out1) -> J_v/1
  p/1 -> Add/1
  pn/1 -> Add/2
  Add/1 -> 3x3 Cross Product/2(In2)
  R/1 -> Product/1
  Constant/1 -> Product/2
  Product/1 -> 3x3 Cross Product/1(In1)

== system ROBOT_OK/Động Lực Học2/Jacobian/J(q) gen./J_v_3(q)/J_v_2/Prismatic Action ==
  R : Inport
  Action Port : ActionPort
  Constant : Constant  Value=[0;0;1]
  Product : Product  Multiplication=Matrix(*)
  J_v : Outport
  wires:
  Product/1 -> J_v/1
  R/1 -> Product/1
  Constant/1 -> Product/2

== system ROBOT_OK/Động Lực Học2/Jacobian/J(q) gen./J_v_3(q)/J_v_2/Revolute Action ==
  R : Inport
  p : Inport  Port=2
  pn : Inport  Port=3
  Action Port : ActionPort
  3x3 Cross Product : Subsystem  Description=Replaced Block  mask(Replaced Block){}
      mask help: This block has been replaced with an empty subsystem because it used functionality that is unavailable in Simulink R2021a.
      mask Display: fprintf('Replaced: %s\n','CrossProduct')
  Add : Sum  Inputs=-+
  Constant : Constant  Value=[0;0;1]
  Product : Product  Multiplication=Matrix(*)
  J_v : Outport
  wires:
  3x3 Cross Product/1(Out1) -> J_v/1
  p/1 -> Add/1
  pn/1 -> Add/2
  Add/1 -> 3x3 Cross Product/2(In2)
  R/1 -> Product/1
  Constant/1 -> Product/2
  Product/1 -> 3x3 Cross Product/1(In1)

== system ROBOT_OK/Động Lực Học2/Jacobian/J(q) gen./J_v_4(q)/J_v_1/Prismatic Action ==
  R : Inport
  Action Port : ActionPort
  Constant : Constant  Value=[0;0;1]
  Product : Product  Multiplication=Matrix(*)
  J_v : Outport
  wires:
  Product/1 -> J_v/1
  R/1 -> Product/1
  Constant/1 -> Product/2

== system ROBOT_OK/Động Lực Học2/Jacobian/J(q) gen./J_v_4(q)/J_v_1/Revolute Action ==
  R : Inport
  p : Inport  Port=2
  pn : Inport  Port=3
  Action Port : ActionPort
  3x3 Cross Product : Subsystem  Description=Replaced Block  mask(Replaced Block){}
      mask help: This block has been replaced with an empty subsystem because it used functionality that is unavailable in Simulink R2021a.
      mask Display: fprintf('Replaced: %s\n','CrossProduct')
  Add : Sum  Inputs=-+
  Constant : Constant  Value=[0;0;1]
  Product : Product  Multiplication=Matrix(*)
  J_v : Outport
  wires:
  3x3 Cross Product/1(Out1) -> J_v/1
  p/1 -> Add/1
  pn/1 -> Add/2
  Add/1 -> 3x3 Cross Product/2(In2)
  R/1 -> Product/1
  Constant/1 -> Product/2
  Product/1 -> 3x3 Cross Product/1(In1)

== system ROBOT_OK/Động Lực Học2/Jacobian/J(q) gen./J_v_4(q)/J_v_2/Prismatic Action ==
  R : Inport
  Action Port : ActionPort
  Constant : Constant  Value=[0;0;1]
  Product : Product  Multiplication=Matrix(*)
  J_v : Outport
  wires:
  Product/1 -> J_v/1
  R/1 -> Product/1
  Constant/1 -> Product/2

== system ROBOT_OK/Động Lực Học2/Jacobian/J(q) gen./J_v_4(q)/J_v_2/Revolute Action ==
  R : Inport
  p : Inport  Port=2
  pn : Inport  Port=3
  Action Port : ActionPort
  3x3 Cross Product : Subsystem  Description=Replaced Block  mask(Replaced Block){}
      mask help: This block has been replaced with an empty subsystem because it used functionality that is unavailable in Simulink R2021a.
      mask Display: fprintf('Replaced: %s\n','CrossProduct')
  Add : Sum  Inputs=-+
  Constant : Constant  Value=[0;0;1]
  Product : Product  Multiplication=Matrix(*)
  J_v : Outport
  wires:
  3x3 Cross Product/1(Out1) -> J_v/1
  p/1 -> Add/1
  pn/1 -> Add/2
  Add/1 -> 3x3 Cross Product/2(In2)
  R/1 -> Product/1
  Constant/1 -> Product/2
  Product/1 -> 3x3 Cross Product/1(In1)

== system ROBOT_OK/Động Lực Học2/Jacobian/J(q) gen./J_v_4(q)/J_v_3/Prismatic Action ==
  R : Inport
  Action Port : ActionPort
  Constant : Constant  Value=[0;0;1]
  Product : Product  Multiplication=Matrix(*)
  J_v : Outport
  wires:
  Product/1 -> J_v/1
  R/1 -> Product/1
  Constant/1 -> Product/2

== system ROBOT_OK/Động Lực Học2/Jacobian/J(q) gen./J_v_4(q)/J_v_3/Revolute Action ==
  R : Inport
  p : Inport  Port=2
  pn : Inport  Port=3
  Action Port : ActionPort
  3x3 Cross Product : Subsystem  Description=Replaced Block  mask(Replaced Block){}
      mask help: This block has been replaced with an empty subsystem because it used functionality that is unavailable in Simulink R2021a.
      mask Display: fprintf('Replaced: %s\n','CrossProduct')
  Add : Sum  Inputs=-+
  Constant : Constant  Value=[0;0;1]
  Product : Product  Multiplication=Matrix(*)
  J_v : Outport
  wires:
  3x3 Cross Product/1(Out1) -> J_v/1
  p/1 -> Add/1
  pn/1 -> Add/2
  Add/1 -> 3x3 Cross Product/2(In2)
  R/1 -> Product/1
  Constant/1 -> Product/2
  Product/1 -> 3x3 Cross Product/1(In1)

== system ROBOT_OK/Động Lực Học2/Jacobian/J(q) gen./J_v_5(q)/J_v_1/Prismatic Action ==
  R : Inport
  Action Port : ActionPort
  Constant : Constant  Value=[0;0;1]
  Product : Product  Multiplication=Matrix(*)
  J_v : Outport
  wires:
  Product/1 -> J_v/1
  R/1 -> Product/1
  Constant/1 -> Product/2

== system ROBOT_OK/Động Lực Học2/Jacobian/J(q) gen./J_v_5(q)/J_v_1/Revolute Action ==
  R : Inport
  p : Inport  Port=2
  pn : Inport  Port=3
  Action Port : ActionPort
  3x3 Cross Product : Subsystem  Description=Replaced Block  mask(Replaced Block){}
      mask help: This block has been replaced with an empty subsystem because it used functionality that is unavailable in Simulink R2021a.
      mask Display: fprintf('Replaced: %s\n','CrossProduct')
  Add : Sum  Inputs=-+
  Constant : Constant  Value=[0;0;1]
  Product : Product  Multiplication=Matrix(*)
  J_v : Outport
  wires:
  3x3 Cross Product/1(Out1) -> J_v/1
  p/1 -> Add/1
  pn/1 -> Add/2
  Add/1 -> 3x3 Cross Product/2(In2)
  R/1 -> Product/1
  Constant/1 -> Product/2
  Product/1 -> 3x3 Cross Product/1(In1)

== system ROBOT_OK/Động Lực Học2/Jacobian/J(q) gen./J_v_5(q)/J_v_2/Prismatic Action ==
  R : Inport
  Action Port : ActionPort
  Constant : Constant  Value=[0;0;1]
  Product : Product  Multiplication=Matrix(*)
  J_v : Outport
  wires:
  Product/1 -> J_v/1
  R/1 -> Product/1
  Constant/1 -> Product/2

== system ROBOT_OK/Động Lực Học2/Jacobian/J(q) gen./J_v_5(q)/J_v_2/Revolute Action ==
  R : Inport
  p : Inport  Port=2
  pn : Inport  Port=3
  Action Port : ActionPort
  3x3 Cross Product : Subsystem  Description=Replaced Block  mask(Replaced Block){}
      mask help: This block has been replaced with an empty subsystem because it used functionality that is unavailable in Simulink R2021a.
      mask Display: fprintf('Replaced: %s\n','CrossProduct')
  Add : Sum  Inputs=-+
  Constant : Constant  Value=[0;0;1]
  Product : Product  Multiplication=Matrix(*)
  J_v : Outport
  wires:
  3x3 Cross Product/1(Out1) -> J_v/1
  p/1 -> Add/1
  pn/1 -> Add/2
  Add/1 -> 3x3 Cross Product/2(In2)
  R/1 -> Product/1
  Constant/1 -> Product/2
  Product/1 -> 3x3 Cross Product/1(In1)

== system ROBOT_OK/Động Lực Học2/Jacobian/J(q) gen./J_v_5(q)/J_v_3/Prismatic Action ==
  R : Inport
  Action Port : ActionPort
  Constant : Constant  Value=[0;0;1]
  Product : Product  Multiplication=Matrix(*)
  J_v : Outport
  wires:
  Product/1 -> J_v/1
  R/1 -> Product/1
  Constant/1 -> Product/2

== system ROBOT_OK/Động Lực Học2/Jacobian/J(q) gen./J_v_5(q)/J_v_3/Revolute Action ==
  R : Inport
  p : Inport  Port=2
  pn : Inport  Port=3
  Action Port : ActionPort
  3x3 Cross Product : Subsystem  Description=Replaced Block  mask(Replaced Block){}
      mask help: This block has been replaced with an empty subsystem because it used functionality that is unavailable in Simulink R2021a.
      mask Display: fprintf('Replaced: %s\n','CrossProduct')
  Add : Sum  Inputs=-+
  Constant : Constant  Value=[0;0;1]
  Product : Product  Multiplication=Matrix(*)
  J_v : Outport
  wires:
  3x3 Cross Product/1(Out1) -> J_v/1
  p/1 -> Add/1
  pn/1 -> Add/2
  Add/1 -> 3x3 Cross Product/2(In2)
  R/1 -> Product/1
  Constant/1 -> Product/2
  Product/1 -> 3x3 Cross Product/1(In1)

== system ROBOT_OK/Động Lực Học2/Jacobian/J(q) gen./J_v_5(q)/J_v_4/Prismatic Action ==
  R : Inport
  Action Port : ActionPort
  Constant : Constant  Value=[0;0;1]
  Product : Product  Multiplication=Matrix(*)
  J_v : Outport
  wires:
  Product/1 -> J_v/1
  R/1 -> Product/1
  Constant/1 -> Product/2

== system ROBOT_OK/Động Lực Học2/Jacobian/J(q) gen./J_v_5(q)/J_v_4/Revolute Action ==
  R : Inport
  p : Inport  Port=2
  pn : Inport  Port=3
  Action Port : ActionPort
  3x3 Cross Product : Subsystem  Description=Replaced Block  mask(Replaced Block){}
      mask help: This block has been replaced with an empty subsystem because it used functionality that is unavailable in Simulink R2021a.
      mask Display: fprintf('Replaced: %s\n','CrossProduct')
  Add : Sum  Inputs=-+
  Constant : Constant  Value=[0;0;1]
  Product : Product  Multiplication=Matrix(*)
  J_v : Outport
  wires:
  3x3 Cross Product/1(Out1) -> J_v/1
  p/1 -> Add/1
  pn/1 -> Add/2
  Add/1 -> 3x3 Cross Product/2(In2)
  R/1 -> Product/1
  Constant/1 -> Product/2
  Product/1 -> 3x3 Cross Product/1(In1)

== system ROBOT_OK/Động Lực Học2/Jacobian/J_v/J_v_1/Revolute Action/3x3 Cross Product ==
  In1 : Inport
  In2 : Inport  Port=2
  Ground1 : Ground
  Terminator1 : Terminator
  Terminator2 : Terminator
  Out1 : Outport
  wires:
  Ground1/1 -> Out1/1
  In2/1 -> Terminator2/1
  In1/1 -> Terminator1/1

== system ROBOT_OK/Động Lực Học2/Jacobian/J_v/J_v_2/Revolute Action/3x3 Cross Product ==
  In1 : Inport
  In2 : Inport  Port=2
  Ground1 : Ground
  Terminator1 : Terminator
  Terminator2 : Terminator
  Out1 : Outport
  wires:
  Ground1/1 -> Out1/1
  In2/1 -> Terminator2/1
  In1/1 -> Terminator1/1

== system ROBOT_OK/Động Lực Học2/Jacobian/J_v/J_v_3/Revolute Action/3x3 Cross Product ==
  In1 : Inport
  In2 : Inport  Port=2
  Ground1 : Ground
  Terminator1 : Terminator
  Terminator2 : Terminator
  Out1 : Outport
  wires:
  Ground1/1 -> Out1/1
  In2/1 -> Terminator2/1
  In1/1 -> Terminator1/1

== system ROBOT_OK/Động Lực Học2/Jacobian/J_v/J_v_4/Revolute Action/3x3 Cross Product ==
  In1 : Inport
  In2 : Inport  Port=2
  Ground1 : Ground
  Terminator1 : Terminator
  Terminator2 : Terminator
  Out1 : Outport
  wires:
  Ground1/1 -> Out1/1
  In2/1 -> Terminator2/1
  In1/1 -> Terminator1/1

== system ROBOT_OK/Động Lực Học2/Jacobian/J_v/J_v_5/Revolute Action/3x3 Cross Product ==
  In1 : Inport
  In2 : Inport  Port=2
  Ground1 : Ground
  Terminator1 : Terminator
  Terminator2 : Terminator
  Out1 : Outport
  wires:
  Ground1/1 -> Out1/1
  In2/1 -> Terminator2/1
  In1/1 -> Terminator1/1

== system ROBOT_OK/Động Lực Học2/Jacobian/J_v/J_v_6/Revolute Action/3x3 Cross Product ==
  In1 : Inport
  In2 : Inport  Port=2
  Ground1 : Ground
  Terminator1 : Terminator
  Terminator2 : Terminator
  Out1 : Outport
  wires:
  Ground1/1 -> Out1/1
  In2/1 -> Terminator2/1
  In1/1 -> Terminator1/1

== system ROBOT_OK/Động Lực Học2/Jacobian/J(q) gen./J_v_2(q)/J_v_1/Revolute Action/3x3 Cross Product ==
  In1 : Inport
  In2 : Inport  Port=2
  Ground1 : Ground
  Terminator1 : Terminator
  Terminator2 : Terminator
  Out1 : Outport
  wires:
  Ground1/1 -> Out1/1
  In2/1 -> Terminator2/1
  In1/1 -> Terminator1/1

== system ROBOT_OK/Động Lực Học2/Jacobian/J(q) gen./J_v_3(q)/J_v_1/Revolute Action/3x3 Cross Product ==
  In1 : Inport
  In2 : Inport  Port=2
  Ground1 : Ground
  Terminator1 : Terminator
  Terminator2 : Terminator
  Out1 : Outport
  wires:
  Ground1/1 -> Out1/1
  In2/1 -> Terminator2/1
  In1/1 -> Terminator1/1

== system ROBOT_OK/Động Lực Học2/Jacobian/J(q) gen./J_v_3(q)/J_v_2/Revolute Action/3x3 Cross Product ==
  In1 : Inport
  In2 : Inport  Port=2
  Ground1 : Ground
  Terminator1 : Terminator
  Terminator2 : Terminator
  Out1 : Outport
  wires:
  Ground1/1 -> Out1/1
  In2/1 -> Terminator2/1
  In1/1 -> Terminator1/1

== system ROBOT_OK/Động Lực Học2/Jacobian/J(q) gen./J_v_4(q)/J_v_1/Revolute Action/3x3 Cross Product ==
  In1 : Inport
  In2 : Inport  Port=2
  Ground1 : Ground
  Terminator1 : Terminator
  Terminator2 : Terminator
  Out1 : Outport
  wires:
  Ground1/1 -> Out1/1
  In2/1 -> Terminator2/1
  In1/1 -> Terminator1/1

== system ROBOT_OK/Động Lực Học2/Jacobian/J(q) gen./J_v_4(q)/J_v_2/Revolute Action/3x3 Cross Product ==
  In1 : Inport
  In2 : Inport  Port=2
  Ground1 : Ground
  Terminator1 : Terminator
  Terminator2 : Terminator
  Out1 : Outport
  wires:
  Ground1/1 -> Out1/1
  In2/1 -> Terminator2/1
  In1/1 -> Terminator1/1

== system ROBOT_OK/Động Lực Học2/Jacobian/J(q) gen./J_v_4(q)/J_v_3/Revolute Action/3x3 Cross Product ==
  In1 : Inport
  In2 : Inport  Port=2
  Ground1 : Ground
  Terminator1 : Terminator
  Terminator2 : Terminator
  Out1 : Outport
  wires:
  Ground1/1 -> Out1/1
  In2/1 -> Terminator2/1
  In1/1 -> Terminator1/1

== system ROBOT_OK/Động Lực Học2/Jacobian/J(q) gen./J_v_5(q)/J_v_1/Revolute Action/3x3 Cross Product ==
  In1 : Inport
  In2 : Inport  Port=2
  Ground1 : Ground
  Terminator1 : Terminator
  Terminator2 : Terminator
  Out1 : Outport
  wires:
  Ground1/1 -> Out1/1
  In2/1 -> Terminator2/1
  In1/1 -> Terminator1/1

== system ROBOT_OK/Động Lực Học2/Jacobian/J(q) gen./J_v_5(q)/J_v_2/Revolute Action/3x3 Cross Product ==
  In1 : Inport
  In2 : Inport  Port=2
  Ground1 : Ground
  Terminator1 : Terminator
  Terminator2 : Terminator
  Out1 : Outport
  wires:
  Ground1/1 -> Out1/1
  In2/1 -> Terminator2/1
  In1/1 -> Terminator1/1

== system ROBOT_OK/Động Lực Học2/Jacobian/J(q) gen./J_v_5(q)/J_v_3/Revolute Action/3x3 Cross Product ==
  In1 : Inport
  In2 : Inport  Port=2
  Ground1 : Ground
  Terminator1 : Terminator
  Terminator2 : Terminator
  Out1 : Outport
  wires:
  Ground1/1 -> Out1/1
  In2/1 -> Terminator2/1
  In1/1 -> Terminator1/1

== system ROBOT_OK/Động Lực Học2/Jacobian/J(q) gen./J_v_5(q)/J_v_4/Revolute Action/3x3 Cross Product ==
  In1 : Inport
  In2 : Inport  Port=2
  Ground1 : Ground
  Terminator1 : Terminator
  Terminator2 : Terminator
  Out1 : Outport
  wires:
  Ground1/1 -> Out1/1
  In2/1 -> Terminator2/1
  In1/1 -> Terminator1/1

== matlab function ROBOT_OK/Động Lực Học2/Jacobian/J_w/v2M_3 ==
  data: v1 input; M output; v2 input
function M = fcn(v1,v2)

M=[v1 v2];

== matlab function ROBOT_OK/Động Lực Học2/Jacobian/J_w/v2M_4 ==
  data: v1 input; M output; v2 input
function M = fcn(v1,v2)

M=[v1 v2];

== matlab function ROBOT_OK/Động Lực Học2/Jacobian/J_w/v2M_5 ==
  data: v1 input; M output; v2 input
function M = fcn(v1,v2)

M=[v1 v2];

== matlab function ROBOT_OK/Động Lực Học2/M(q),C(q,dq),g(q)/M,H/MATLAB Function ==
  data: m input; M output; I1 input; I2 input; I3 input; I4 input; I5 input; I6 input; W1 input; W2 input; W3 input; W4 input; W5 input; W6 input; H output
function [M,H] = fcn(m,I1,I2,I3,I4,I5,I6,W1,W2,W3,W4,W5,W6)
%#codegen

M = blkdiag(m(1)*eye(3),m(2)*eye(3),m(3)*eye(3),m(4)*eye(3),m(5)*eye(3),m(6)*eye(3),...
            I1,I2,I3,I4,I5,I6);

H =-blkdiag(zeros(18,18),W1,W2,W3,W4,W5,W6);

== matlab function ROBOT_OK/Subsystem2/Jacobian/J(q) gen./J_v_1(q)/v2M_1 ==
  data: v1 input; M output; v2 input
function M = fcn(v1,v2)

M=[v1 v2];
